simulink model "Optitrack_Simulink_TrackableLocation"  (R2014a)
settings: Solver=ode5  StartTime=0.0  StopTime=inf  RelTol=1e-3
settings Model: Creator=sasson  LastModifiedBy=sasson
settings HardwareCC: ProdIntDivRoundTo=Zero  ProdEndianess=LittleEndian  ProdHWDeviceType=Generic->32-bit x86 compatible
settings RTWCC: SystemTargetFile=rtwin.tlc  TemplateMakefile=rtwin.tmf  Description=Real-Time Windows Target  ProcessScript=rtwin_make_rtw_hook  TargetLang=C++  RTWCompilerOptimization=On
settings CodeAppCC: MaxIdLength=95
settings RTWinTargetCC: TargetLibSuffix=_rtwin.lib  TargetPreCompLibLocation=C:\Program Files\MATLAB\R2014a\toolbox\rtw\targets\rtwin\lib\win64

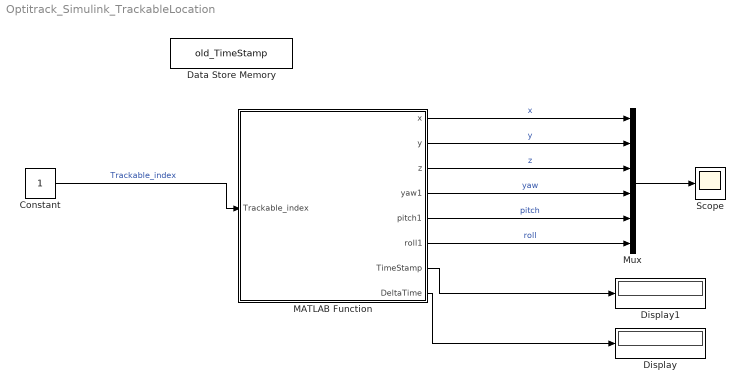
== system Optitrack_Simulink_TrackableLocation ==
  Constant : Constant  OutDataTypeStr=Inherit: Inherit via back propagation
  Data Store Memory : DataStoreMemory  DataStoreName=old_TimeStamp  ReadBeforeWriteMsg=warning  WriteAfterWriteMsg=warning  WriteAfterReadMsg=warning  OutDataTypeStr=double
  Display : Display
  Display1 : Display
  MATLAB Function : MATLAB Function  TreatAsAtomicUnit=on
  Mux : Mux  Inputs=6
  Scope : Scope
  wires:
  Constant/1 -> MATLAB Function/1(Trackable_index)  "Trackable_index"
  Mux/1 -> Scope/1
  MATLAB Function/6(roll1) -> Mux/6  "roll"
  MATLAB Function/5(pitch1) -> Mux/5  "pitch"
  MATLAB Function/4(yaw1) -> Mux/4  "yaw"
  MATLAB Function/3(z) -> Mux/3  "z"
  MATLAB Function/2(y) -> Mux/2  "y"
  MATLAB Function/1(x) -> Mux/1  "x"
  MATLAB Function/7(TimeStamp) -> Display1/1
  MATLAB Function/8(DeltaTime) -> Display/1

== matlab function Optitrack_Simulink_TrackableLocation/MATLAB Function ==
  data: Trackable_index input; x output; y output; z output; yaw1 output; pitch1 output; roll1 output; TimeStamp output; DeltaTime output; old_TimeStamp data_store_memory
function [x,y,z,yaw1,pitch1,roll1,TimeStamp,DeltaTime]=TrackableLocation(Trackable_index)
    coder.extrinsic('calllib') % define matlab function in simulink
    
    global old_TimeStamp
    
    %update frame
    calllib('NPTrackingTools', 'TT_UpdateSingleFrame'); %refresh data
   
    %define the outputs types from TT_TrackableLocation function
    %for the function it's need to be single data type
    X=single(0);Y=single(0);Z=single(0);
    yaw=single(0); pitch=single(0); roll=single(0);
    qx=single(0);qy=single(0);qz=single(0);qw=single(0);
    TimeStamp1=double(0);
    
    % find the location of any trackable
    [X,Y,Z,qx,qy,qz,qw,yaw,pitch,roll] = calllib('NPTrackingTools', 'TT_TrackableLocation',(Trackable_index-1),X,Y,Z,qx,qy,qz,qw,yaw,pitch,roll);
    TimeStamp1 = calllib('NPTrackingTools', 'TT_FrameTimeStamp');
    
    % simulink accept only double data type
    x=double(X); y=double(Y); z=double(Z);
    yaw1=double(yaw); pitch1=double(pitch); roll1=double(roll);
    TimeStamp=double(TimeStamp1);
    
    
    DeltaTime=TimeStamp-old_TimeStamp;
    old_TimeStamp=TimeStamp;
end
